simulink model "can_observer_org"  (Simulink 10.0)
settings: Solver=ode45  StartTime=0.0  StopTime=20  RelTol=1e-3  EnableMultiTasking=on
InitFcn:
  | param
undefined symbols (not defined in the file): can_ctrl, P
libraries: simulink x1
settings Model: Creator=paul  LastModifiedBy=annonymous
settings DataIOCC: LimitDataPoints=on
settings DebuggingCC: SolverPrmCheckMsg=warning
settings GRTTargetCC: GeneratePreprocessorConditionals=Disable all  CombineOutputUpdateFcns=on  GRTInterface=off
settings ConfigComp: CovExternalEMLEnable=off

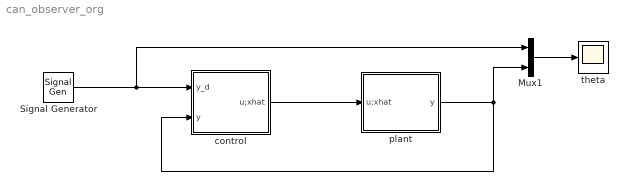
== system can_observer_org ==
  Mux1 : Mux  Inputs=2
  Signal Generator : SignalGenerator  WaveForm=square  Amplitude=2  Units=rad/sec
  control : Subsystem
  plant : Subsystem
  theta : Scope
  wires:
  Signal Generator/1 -> control/1(y_d), Mux1/1
  Mux1/1 -> theta/1
  plant/1(y) -> control/2(y), Mux1/2
  control/1(u;xhat) -> plant/1(u;xhat)

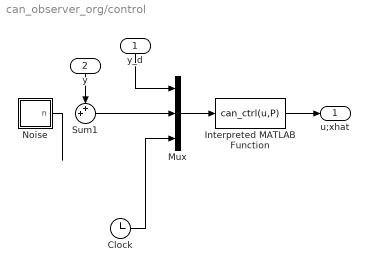
== system can_observer_org/control ==
  y_d : Inport
  y : Inport  Port=2
  Clock : Clock
  Interpreted MATLAB Function : MATLABFcn  MATLABFcn=can_ctrl(u,P)  OutputDimensions=1+2  SampleTime=P.Ts
  Mux : Mux  Inputs=3
  Noise : Subsystem
  Sum1 : Sum  Inputs=++|
  u;xhat : Outport
  wires:
  Noise/1(n) -> ?
  Interpreted MATLAB Function/1 -> u;xhat/1
  y/1 -> Sum1/1
  Sum1/1 -> Mux/2
  y_d/1 -> Mux/1
  Mux/1 -> Interpreted MATLAB Function/1
  Clock/1 -> Mux/3

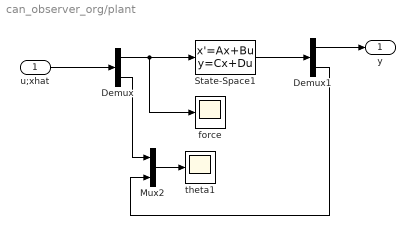
== system can_observer_org/plant ==
  u;xhat : Inport
  Demux : Demux  Outputs=2
  Demux1 : Demux  Outputs=2
  Mux2 : Mux  Inputs=2
  State-Space1 : StateSpace  A=P.A  B=P.B  C=[P.C; eye(2)]  D=[P.D; 0; 0]  InitialCondition=[0;0]
  force : Scope
  theta1 : Scope
  y : Outport
  wires:
  Demux1/1 -> y/1
  State-Space1/1 -> Demux1/1
  u;xhat/1 -> Demux/1
  Mux2/1 -> theta1/1
  Demux/2 -> Mux2/1
  Demux/1 -> force/1, State-Space1/1
  Demux1/2 -> Mux2/2

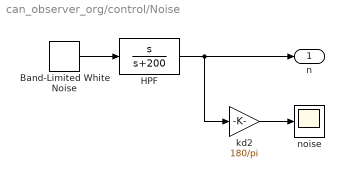
== system can_observer_org/control/Noise ==
  Band-Limited White Noise : simulink/Sources/Band-Limited White Noise  Cov=[0.0001]  Ts=P.Ts  seed=[23341]
  HPF : TransferFcn  Numerator=[1 0]  Denominator=[1 200]
  kd2 : Gain  Gain=180/pi
  noise : Scope
  n : Outport
  wires:
  Band-Limited White Noise/1 -> HPF/1
  kd2/1 -> noise/1
  HPF/1 -> kd2/1, n/1
